simulink model "fcw"  (R2026a)
settings: Solver=FixedStepDiscrete  StopTime=300  FixedStep=Tsmp  EnableMultiTasking=on
InitFcn:
  | tp_min=0.3;
  | tp_max=0.75;
  | W=1125;
  | g=9.81;
  | rho=1.18;
  | Af=2.63;
  | Cd=0.32;
  | gamma=1.04;
  | fr=0.015;
  | Tc=2.5;
  | Cae=0.497;
  | u_min=0.75;
  | u_max=0.9;
  | nb_min=0.85;
  | nb_max=0.95;
  | age=20;
  | Tsmp=0.001;
  | Td=1;
settings Model: CodeVerificationMode=processor-in-the-loop (pil)  SnapshotBufferSize=100  SnapshotInterval=2  PacingRate=0.100000  LastModifiedBy=Swpnil
settings DataIOCC: ExternalInput=Sheet1.getElement('V'),Sheet1.getElement('theta_s'),Sheet1.getElement('D')  MaxDataPoints=10000000  LoadExternalInput=on  LoggingFileName=yo.mat
settings OptimizationCC: UseDivisionForNetSlopeComputation=on  GainParamInheritBuiltInType=on  UseFloatMulNetSlope=on  InlineInvariantSignals=on  NoFixptDivByZeroProtection=on  EfficientFloat2IntCast=on  LifeSpan=1  MaxStackSize=512
settings DebuggingCC: UnderSpecifiedDimensionMsg=warning
settings HardwareCC: ProdLargestAtomicInteger=Long  ProdLargestAtomicFloat=Double  ProdHWDeviceType=ARM Compatible->ARM Cortex-M
settings RTWCC: SystemTargetFile=ert.tlc  HardwareBoard=STM32F4xx Based  TLCOptions=-aInlineSetEventsForThisBaseRateFcn=TLC_FALSE -aSuppressMultiTaskScheduler=TLC_FALSE -aRateBasedStepFcn=1  Toolchain=GNU Tools for STM32  PortableWordSizes=on  CreateSILPILBlock=PIL  Description=Embedded Coder
settings CodeAppCC: CustomSymbolStrGlobalVar=rt$N$M  CustomSymbolStrType=$N$M  CustomSymbolStrFcn=$N$M$F  CustomSymbolStrMacro=$N$M
settings ERTTargetCC: ExtModeTransport=3.0  ExtModeStaticAllocSize=2048.0  ERTFilePackagingFormat=CompactWithDataFile  CodeReplacementLibrary=ARM Cortex-M  IncludeMdlTerminateFcn=off  CombineSignalStateStructs=on  SupportAbsoluteTime=off  SupportComplex=off  SupportNonInlinedSFcns=on

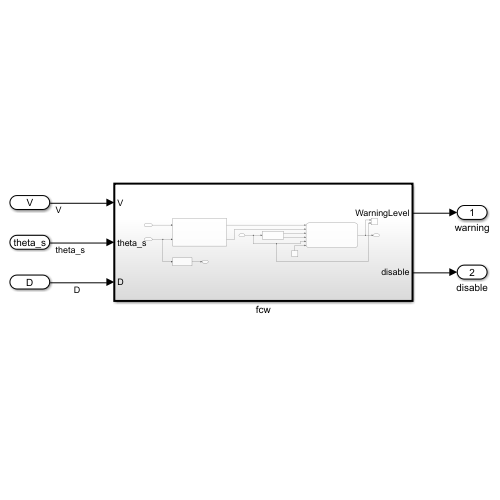
[thumbnail: Simulink's stored preview of the top-level diagram]
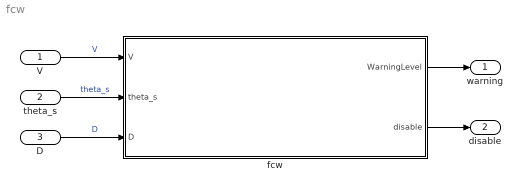
== system fcw ==
  V : Inport  OutDataTypeStr=double  PortDimensions=1  Interpolate=off
  theta_s : Inport  Port=2  OutDataTypeStr=double  PortDimensions=1  Interpolate=off
  D : Inport  Port=3  OutDataTypeStr=double  PortDimensions=1  Interpolate=off
  fcw : Subsystem  TreatAsAtomicUnit=on
  warning : Outport
  disable : Outport  Port=2
  wires:
  theta_s/1 -> fcw/2(theta_s)  "theta_s"
  D/1 -> fcw/3(D)  "D"
  V/1 -> fcw/1(V)  "V"
  fcw/1(WarningLevel) -> warning/1
  fcw/2(disable) -> disable/1

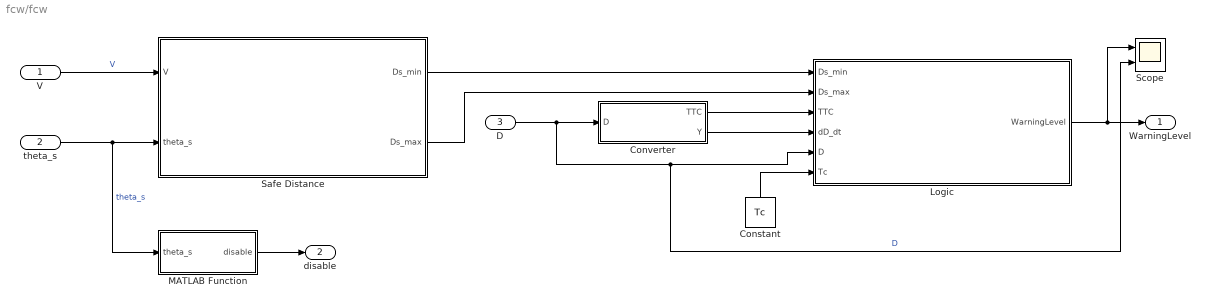
== system fcw/fcw ==
  V : Inport  OutDataTypeStr=double  PortDimensions=1  Interpolate=off
  theta_s : Inport  Port=2  OutDataTypeStr=double  PortDimensions=1  Interpolate=off
  D : Inport  Port=3  OutDataTypeStr=double  PortDimensions=1  Interpolate=off
  Constant : Constant  Value=Tc
  Converter : Subsystem
  Logic : Stateflow chart  TreatAsAtomicUnit=on  SystemSampleTime=Tsmp
      settings: PortSchema="{\"entries\":[{\"content\":{\"sides\":[{\"content\":{\"connectorIds\":[\"In1\",\"In2\",\"In3\",\"In6\",\"In4\",\"In5\"]},\"type\":\"ConnectorPlacement.EquallySpacedRectSide\",\"uuid\":\"1c1c9de1-d4de-4feb-957b-a8329dc61873\"},{\"content\":{\"connectorIds\":[\"Out1\"],\"side\":\"RIGHT\"},\"type\":\"ConnectorPlacement.EquallySpacedRectSide\",\"uuid\":\"0311181c-176b-4e74-867f-e9bb057240a0\"},{\"content\":{\"side\":\"TOP\"},\"type\":\"ConnectorPlacement.EquallySpacedRectSide\",\"uuid\":\"c507be71-833c-42c3-bbab-a1cda7bc9fec\"}]},\"type\":\"ConnectorPlacement.EquallySpacedConnector\",\"uuid\":\"347675f7-d269-449f-95d4-f0d43ee2fcf2\"}],\"packageUris\":[\"http://schema.mathworks.com/mf0/Connector/R2020b\"],\"version\":\"1.0\"}"
  MATLAB Function : MATLAB Function  TreatAsAtomicUnit=on
  Safe Distance : Subsystem
  Scope : Scope  NumInputPorts=2
      settings: ActiveDisplayYMinimum=0.98139464111587937  ActiveDisplayYMaximum=1.118314810169184
  WarningLevel : Outport  OutDataTypeStr=uint64
  disable : Outport  Port=2
  wires:
  Converter/2(Y) -> Logic/6(dD_dt)
  Constant/1 -> Logic/5(Tc)
  Converter/1(TTC) -> Logic/3(TTC)
  Safe Distance/2(Ds_max) -> Logic/2(Ds_max)
  V/1 -> Safe Distance/1(V)  "V"
  D/1 -> Scope/2, Logic/4(D), Converter/1(D)  "D"
  Safe Distance/1(Ds_min) -> Logic/1(Ds_min)
  theta_s/1 -> MATLAB Function/1(theta_s), Safe Distance/2(theta_s)  "theta_s"
  Logic/1(WarningLevel) -> Scope/1, WarningLevel/1
  MATLAB Function/1(disable) -> disable/1

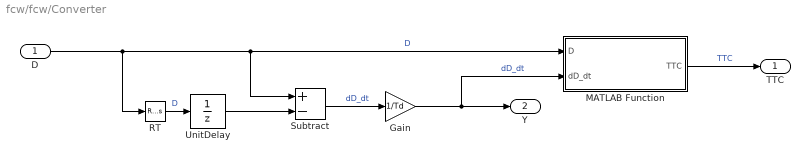
== system fcw/fcw/Converter ==
  D : Inport  OutDataTypeStr=double
  Gain : Gain  Gain=1/Td
  MATLAB Function : MATLAB Function  TreatAsAtomicUnit=on
  RT : RateTransition  Deterministic=off  OutPortSampleTime=Td
  Subtract : Sum  Inputs=+-
  UnitDelay : UnitDelay  SampleTime=Td
  TTC : Outport  OutDataTypeStr=double
  Y : Outport  Port=2  OutDataTypeStr=double
  wires:
  D/1 -> RT/1, Subtract/1, MATLAB Function/1(D)  "D"
  MATLAB Function/1(TTC) -> TTC/1  "TTC"
  Subtract/1 -> Gain/1  "dD_dt"
  RT/1 -> UnitDelay/1  "D"
  Gain/1 -> MATLAB Function/2(dD_dt), Y/1  "dD_dt"
  UnitDelay/1 -> Subtract/2

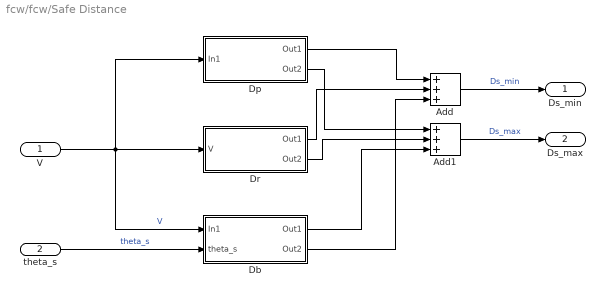
== system fcw/fcw/Safe Distance ==
  V : Inport
  theta_s : Inport  Port=2
  Add : Sum  Inputs=+++
  Add1 : Sum  Inputs=+++
  Db : Subsystem
  Dp : Subsystem
  Dr : Subsystem
  Ds_min : Outport
  Ds_max : Outport  Port=2
  wires:
  Db/2(Out2) -> Add/3
  Db/1(Out1) -> Add1/3
  Dp/1(Out1) -> Add/1
  Dr/2(Out2) -> Add1/2
  Dp/2(Out2) -> Add1/1
  theta_s/1 -> Db/2(theta_s)  "theta_s"
  Dr/1(Out1) -> Add/2
  V/1 -> Dr/1(V), Db/1(In1), Dp/1(In1)  "V"
  Add/1 -> Ds_min/1  "Ds_min"
  Add1/1 -> Ds_max/1  "Ds_max"

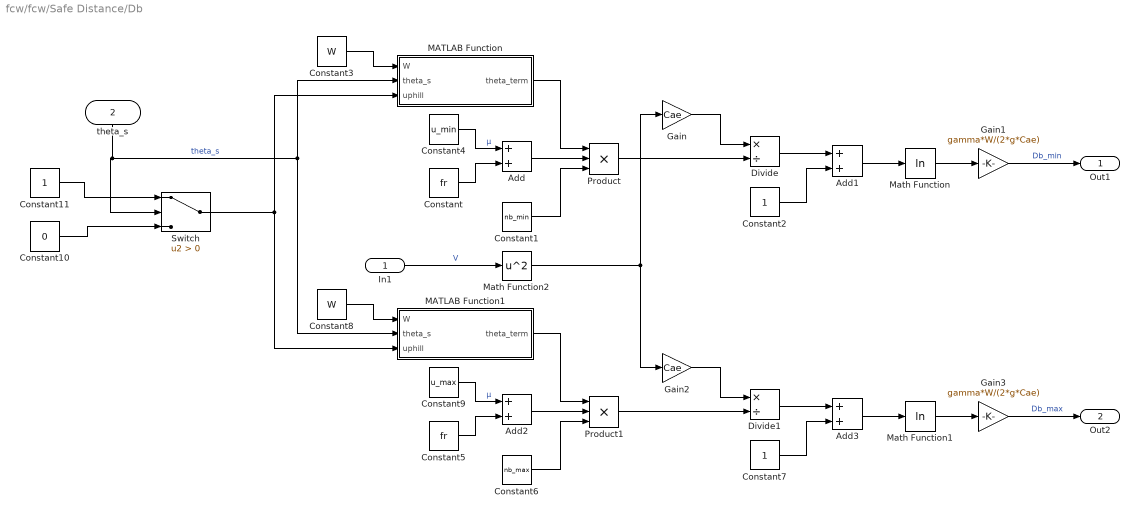
== system fcw/fcw/Safe Distance/Db ==
  In1 : Inport
  theta_s : Inport  Port=2
  Add{,1..3} (4 alike) : Sum
  Constant : Constant  Value=fr
  Constant1 : Constant  Value=nb_min
  Constant10 : Constant  Value=0  OutDataTypeStr=boolean
  Constant11 : Constant  OutDataTypeStr=boolean
  Constant2 : Constant
  Constant3 : Constant  Value=W
  Constant4 : Constant  Value=u_min
  Constant5 : Constant  Value=fr
  Constant6 : Constant  Value=nb_max
  Constant7 : Constant
  Constant8 : Constant  Value=W
  Constant9 : Constant  Value=u_max
  Divide : Product  Inputs=*/
  Divide1 : Product  Inputs=*/
  Gain : Gain  Gain=Cae
  Gain1 : Gain  Gain=gamma*W/(2*g*Cae)
  Gain2 : Gain  Gain=Cae
  Gain3 : Gain  Gain=gamma*W/(2*g*Cae)
  MATLAB Function : MATLAB Function  TreatAsAtomicUnit=on
  MATLAB Function1 : MATLAB Function  TreatAsAtomicUnit=on
  Math Function : Math  Operator=log
  Math Function1 : Math  Operator=log
  Math Function2 : Math  Operator=square
  Product : Product  Inputs=3
  Product1 : Product  Inputs=3
  Switch : Switch  Criteria=u2 > Threshold  SaturateOnIntegerOverflow=off  InputSameDT=off
  Out1 : Outport
  Out2 : Outport  Port=2
  wires:
  Constant4/1 -> Add/1  "μ"
  Constant/1 -> Add/2
  Add/1 -> Product/2
  MATLAB Function/1(theta_term) -> Product/1
  Constant1/1 -> Product/3
  Product/1 -> Divide/2
  Gain/1 -> Divide/1
  Divide/1 -> Add1/1
  Constant2/1 -> Add1/2
  Add1/1 -> Math Function/1
  Math Function/1 -> Gain1/1
  Constant3/1 -> MATLAB Function/1(W)
  Add3/1 -> Math Function1/1
  MATLAB Function1/1(theta_term) -> Product1/1
  Gain2/1 -> Divide1/1
  Constant9/1 -> Add2/1  "μ"
  Switch/1 -> MATLAB Function/3(uphill), MATLAB Function1/3(uphill)
  Divide1/1 -> Add3/1
  Constant6/1 -> Product1/3
  Constant7/1 -> Add3/2
  Add2/1 -> Product1/2
  Constant5/1 -> Add2/2
  Constant8/1 -> MATLAB Function1/1(W)
  Product1/1 -> Divide1/2
  Math Function1/1 -> Gain3/1
  Gain3/1 -> Out2/1  "Db_max"
  Gain1/1 -> Out1/1  "Db_min"
  In1/1 -> Math Function2/1  "V"
  theta_s/1 -> Switch/2, MATLAB Function1/2(theta_s), MATLAB Function/2(theta_s)  "theta_s"
  Constant11/1 -> Switch/1
  Constant10/1 -> Switch/3
  Math Function2/1 -> Gain2/1, Gain/1

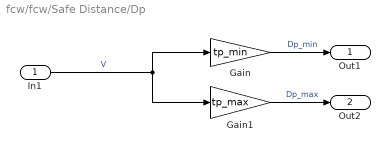
== system fcw/fcw/Safe Distance/Dp ==
  In1 : Inport
  Gain : Gain  Gain=tp_min
  Gain1 : Gain  Gain=tp_max
  Out1 : Outport
  Out2 : Outport  Port=2
  wires:
  Gain/1 -> Out1/1  "Dp_min"
  Gain1/1 -> Out2/1  "Dp_max"
  In1/1 -> Gain1/1, Gain/1  "V"

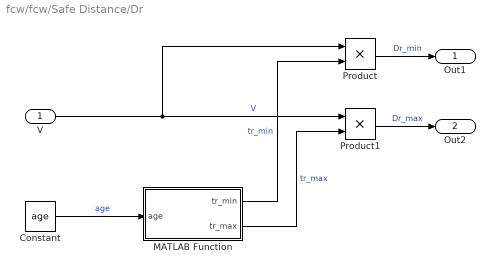
== system fcw/fcw/Safe Distance/Dr ==
  V : Inport
  Constant : Constant  Value=age
  MATLAB Function : MATLAB Function  TreatAsAtomicUnit=on
  Product : Product
  Product1 : Product
  Out1 : Outport
  Out2 : Outport  Port=2
  wires:
  Product/1 -> Out1/1  "Dr_min"
  Product1/1 -> Out2/1  "Dr_max"
  MATLAB Function/1(tr_min) -> Product/2  "tr_min"
  MATLAB Function/2(tr_max) -> Product1/2  "tr_max"
  Constant/1 -> MATLAB Function/1(age)  "age"
  V/1 -> Product/1, Product1/1  "V"

== matlab function fcw/Safe Distance/Db/MATLAB Function ==
  data: W input; theta_term output; theta_s input; uphill input
function theta_term = roadSlopeTerm(W, theta_s, uphill)


    if uphill==1
        theta_term = W*cosd(theta_s) + W*sind(theta_s);
    else
        theta_term = W*cosd(theta_s) - W*sind(theta_s);
    end
end

== matlab function fcw/Safe Distance/Dr/MATLAB Function ==
  data: age input; tr_min output; tr_max output
function [tr_min, tr_max] = getTr(age)

if age >= 18 && age <= 33
    tr_min = 0.74;
    tr_max = 1.10;

elseif age <= 47
    tr_min = 0.75;
    tr_max = 1.12;

elseif age <= 57
    tr_min = 0.77;
    tr_max = 1.13;

elseif age <= 70
    tr_min = 0.78;
    tr_max = 1.17;

else
    % Default
    tr_min = 0.78;
    tr_max = 1.17;
end

== stateflow chart fcw/Logic ==
  state decision
  state rule1
    state Level_3_Dangerous
      entry:
      WarningLevel = 3;
    state Rule1
    state Level_1_Warning
      entry:
      WarningLevel = 1;
    state Level_2_Warning
      entry:
      WarningLevel = 2;
    (default) -> Rule1
    Rule1 -> Level_3_Dangerous [order 1] : [TTC < Tc]
    Rule1 -> rule1.Level_1_Warning [order 3] : [TTC >= Tc && dD_dt > 0]
    Level_3_Dangerous -> 197 [order 1] : [D>=Ds_min]
    rule1.Level_1_Warning -> Rule1 [order 2] : [TTC < Tc || dD_dt <= 0]
    (junction 194) -> 197
    Level_3_Dangerous -> Rule1 [order 2] : [TTC >= Tc]
    rule1.Level_1_Warning -> (junction 196) [order 1] : [D>=Ds_min]
    Rule1 -> Level_2_Warning [order 2] : [TTC >= Tc && dD_dt <= 0]
    Level_2_Warning -> Rule1 [order 2] : [TTC < Tc || dD_dt > 0]
    Level_2_Warning -> (junction 194) [order 1] : [D>=Ds_min]
    (junction 195) -> (junction 194)
    (junction 196) -> (junction 195)
  state rule2
    state Level_2_Dangerous
      entry:
      WarningLevel = 2;
    state Rule2
    state Level_0_Warning
      entry:
      WarningLevel = 0;
    state Level_1_Warning
      entry:
      WarningLevel = 1;
    (default) -> Rule2
    Rule2 -> Level_2_Dangerous [order 1] : [TTC < Tc]
    Rule2 -> Level_0_Warning [order 3] : [TTC >= Tc && dD_dt > 0]
    Level_2_Dangerous -> 224 [order 1] : [D>=Ds_max || D<Ds_min]
    (junction 221) -> 224
    Level_0_Warning -> Rule2 [order 2] : [TTC < Tc || dD_dt <= 0]
    Level_2_Dangerous -> Rule2 [order 2] : [TTC >= Tc]
    Rule2 -> rule2.Level_1_Warning [order 2] : [TTC >= Tc && dD_dt <= 0]
    rule2.Level_1_Warning -> Rule2 [order 2] : [TTC < Tc || dD_dt > 0]
    Level_0_Warning -> (junction 223) [order 1] : [D>=Ds_max || D<Ds_min]
    rule2.Level_1_Warning -> (junction 221) [order 1] : [D>=Ds_max || D<Ds_min]
    (junction 222) -> (junction 221)
    (junction 223) -> (junction 222)
  state safeDriving
    entry:
    WarningLevel=5;
  note: Exit
  (default) -> decision
  (junction 244) -> decision
  (junction 242) -> (junction 244)
  decision -> (junction 33)
  (junction 33) -> rule1 [order 1] : [D<Ds_min]{rule=1;}
  192 -> (junction 242)
  (junction 33) -> (junction 38) [order 2]
  (junction 243) -> (junction 242)
  219 -> (junction 243)
  (junction 38) -> rule2 [order 1] : [D<Ds_max]{rule=2;}
  (junction 251) -> (junction 243)
  (junction 38) -> safeDriving [order 2] : {rule=5;}
  safeDriving -> (junction 251) : [D<Ds_max]
  data: Ds_min input; Ds_max input; TTC input; D input; Tc input; dD_dt input; WarningLevel output; rule local

== matlab function fcw/Safe Distance/Db/MATLAB Function1 ==
  data: W input; theta_term output; theta_s input; uphill input
function theta_term = roadSlopeTerm(W, theta_s, uphill)


    if uphill==1
        theta_term = W*cosd(theta_s) + W*sind(theta_s);
    else
        theta_term = W*cosd(theta_s) - W*sind(theta_s);
    end
end

== matlab function fcw/Converter/MATLAB Function ==
  data: D input; TTC output; dD_dt input
function TTC = calcTTC(D,dD_dt)

if abs(dD_dt) < 0.01
    TTC = 999;
else
    TTC = D/abs(dD_dt);
end

end

== matlab function fcw/MATLAB Function ==
  data: theta_s input; disable output
function disable = fcn(theta_s)

% If theta_s is in degrees
if abs(theta_s) > 60
    disable = 1;      % Disable FCW
else
    disable = 0;
end

end
